simulink library "csu_dsm_dsmac_lib"  (R2014b)
settings: Solver=ode45  SolverMode=SingleTasking  StartTime=0.0  StopTime=10.0  RelTol=1e-3
undefined symbols (not defined in the file): rdr_range_max
libraries: simulink x5, util_common_lib x1
settings Model: Creator=eleanor  LastModifiedBy=mstewart

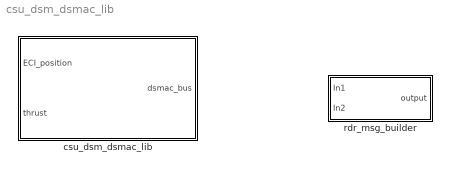
== system csu_dsm_dsmac_lib ==
  csu_dsm_dsmac_lib : Subsystem  SystemSampleTime=0.1
  rdr_msg_builder : Subsystem

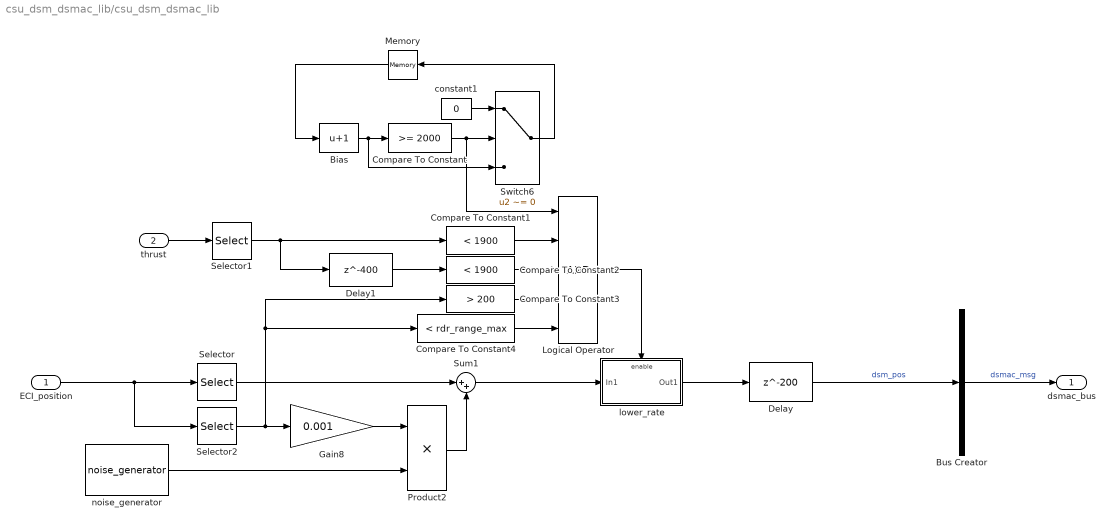
== system csu_dsm_dsmac_lib/csu_dsm_dsmac_lib ==
  ECI_position : Inport
  thrust : Inport  Port=2
  Bias : Bias  Bias=1
  Bus Creator : BusCreator  Inputs=1  OutDataTypeStr=Bus: dsmac_msg  NonVirtualBus=on
  Compare To Constant : simulink/Logic and Bit Operations/Compare To Constant  relop=>=  const=2000  OutDataTypeStr=uint8
  Compare To Constant1 : simulink/Logic and Bit Operations/Compare To Constant  relop=<  const=1900  OutDataTypeStr=uint8
  Compare To Constant2 : simulink/Logic and Bit Operations/Compare To Constant  relop=<  const=1900  OutDataTypeStr=uint8
  Compare To Constant3 : simulink/Logic and Bit Operations/Compare To Constant  relop=>  const=200  OutDataTypeStr=uint8
  Compare To Constant4 : simulink/Logic and Bit Operations/Compare To Constant  relop=<  const=rdr_range_max  OutDataTypeStr=uint8
  Delay : Delay  DelayLength=200
  Delay1 : Delay  DelayLength=400
  Gain8 : Gain  Gain=0.001
  Logical Operator : Logic  Inputs=5  AllPortsSameDT=off  OutDataTypeStr=boolean
  Memory : Memory  X0=799  InheritSampleTime=on
  Product2 : Product  RndMeth=Zero
  Selector : Selector  InputPortWidth=3  Indices=[1 2]
  Selector1 : Selector  InputPortWidth=3  Indices=[3]
  Selector2 : Selector  InputPortWidth=3  Indices=[3]
  Sum1 : Sum  Inputs=|++
  Switch6 : Switch  Criteria=u2 ~= 0  InputSameDT=on
  constant1 : Constant  Value=0
  lower_rate : Subsystem  TreatAsAtomicUnit=on
  noise_generator : util_common_lib/noise_generator  std_dev=1  bias=0  seed=1  on=1  sample_time=sim_time_step_size
  dsmac_bus : Outport
  wires:
  Compare To Constant3/1 -> Logical Operator/4
  Product2/1 -> Sum1/2
  noise_generator/1 -> Product2/2
  Gain8/1 -> Product2/1
  Selector2/1 -> Gain8/1, Compare To Constant3/1, Compare To Constant4/1
  Compare To Constant2/1 -> Logical Operator/3
  Delay1/1 -> Compare To Constant2/1
  Logical Operator/1 -> lower_rate/Enable
  Compare To Constant1/1 -> Logical Operator/2
  Selector1/1 -> Delay1/1, Compare To Constant1/1
  thrust/1 -> Selector1/1
  Memory/1 -> Bias/1
  Switch6/1 -> Memory/1
  Compare To Constant/1 -> Logical Operator/1, Switch6/2
  Bias/1 -> Switch6/3, Compare To Constant/1
  constant1/1 -> Switch6/1
  lower_rate/1(Out1) -> Delay/1
  Bus Creator/1 -> dsmac_bus/1  "dsmac_msg"
  ECI_position/1 -> Selector2/1, Selector/1
  Selector/1 -> Sum1/1
  Sum1/1 -> lower_rate/1(In1)
  Delay/1 -> Bus Creator/1  "dsm_pos"
  Compare To Constant4/1 -> Logical Operator/5

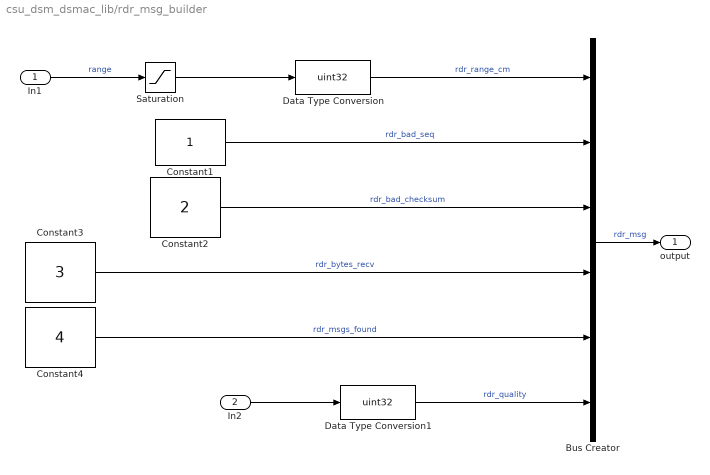
== system csu_dsm_dsmac_lib/rdr_msg_builder ==
  In1 : Inport
  In2 : Inport  Port=2
  Bus Creator : BusCreator  Inputs='rdr_range_cm','rdr_bad_seq','rdr_bad_checksum','rdr_bytes_recv','rdr_msgs_found','rdr_quality'
  Constant1 : Constant  OutDataTypeStr=uint32
  Constant2 : Constant  Value=2  OutDataTypeStr=uint32
  Constant3 : Constant  Value=3  OutDataTypeStr=uint32
  Constant4 : Constant  Value=4  OutDataTypeStr=uint32
  Data Type Conversion : DataTypeConversion  OutDataTypeStr=uint32  SaturateOnIntegerOverflow=on
  Data Type Conversion1 : DataTypeConversion  OutDataTypeStr=uint32  SaturateOnIntegerOverflow=on
  Saturation : Saturate  UpperLimit=4.2950e+009  LowerLimit=0
  output : Outport
  wires:
  In2/1 -> Data Type Conversion1/1
  Data Type Conversion1/1 -> Bus Creator/6  "rdr_quality"
  Constant4/1 -> Bus Creator/5  "rdr_msgs_found"
  Constant3/1 -> Bus Creator/4  "rdr_bytes_recv"
  Constant2/1 -> Bus Creator/3  "rdr_bad_checksum"
  Constant1/1 -> Bus Creator/2  "rdr_bad_seq"
  Bus Creator/1 -> output/1  "rdr_msg"
  Data Type Conversion/1 -> Bus Creator/1  "rdr_range_cm"
  In1/1 -> Saturation/1  "range"
  Saturation/1 -> Data Type Conversion/1

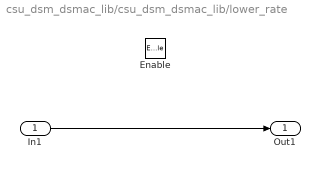
== system csu_dsm_dsmac_lib/csu_dsm_dsmac_lib/lower_rate ==
  In1 : Inport
  Enable : EnablePort
  Out1 : Outport
  wires:
  In1/1 -> Out1/1
